simulink library "udp_library"  (Simulink 7.5)
settings: Solver=ode45  StartTime=0.0  StopTime=10.0  RelTol=1e-3
InitFcn:
  | updateAnnotation.m
undefined symbols (not defined in the file): updateAnnotation
settings Model: Creator=paul  LastModifiedBy=paul.liu

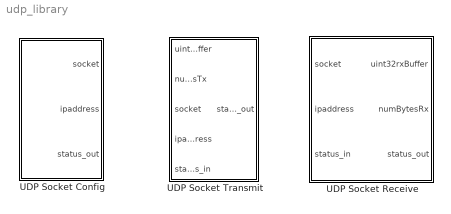
== system udp_library ==
  UDP Socket Config : Subsystem  InitFcn=updateAnnotation();  mask{server_ip='127.0.0.1', server_port=1002, client_ip='127.0.0.1', client_port=1001}
      mask prompts: server_ip "Server IP"; server_port "Server Port"; client_ip "Client IP"; client_port "Client Port"
      settings: AttributesFormatString=Ver 1.0
  UDP Socket Receive : Subsystem  InitFcn=updateAnnotation();
      settings: AttributesFormatString=Ver 1.0
  UDP Socket Transmit : Subsystem  InitFcn=updateAnnotation();
      settings: AttributesFormatString=Ver 1.0

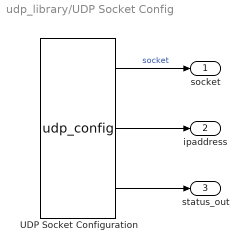
== system udp_library/UDP Socket Config ==
  UDP Socket Configuration : S-Function  FunctionName=udp_config  Parameters=server_ip,server_port,client_ip,client_port  EnableBusSupport=off
  socket : Outport  OutDataType=fixdt(1, 16)  OutScaling=2^0
  ipaddress : Outport  Port=2  OutDataType=fixdt(1, 16)  OutScaling=2^0
  status_out : Outport  Port=3  OutDataType=fixdt(1, 16)  OutScaling=2^0
  wires:
  UDP Socket Configuration/1 -> socket/1  "socket"
  UDP Socket Configuration/2 -> ipaddress/1
  UDP Socket Configuration/3 -> status_out/1

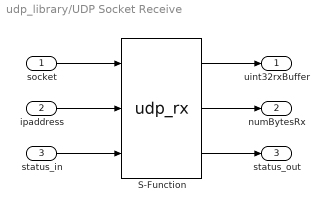
== system udp_library/UDP Socket Receive ==
  socket : Inport  OutDataType=fixdt(1, 16)  OutScaling=2^0
  ipaddress : Inport  Port=2  OutDataType=fixdt(1, 16)  OutScaling=2^0
  status_in : Inport  Port=3  OutDataType=fixdt(1, 16)  OutScaling=2^0
  S-Function : S-Function  FunctionName=udp_rx  EnableBusSupport=off
  uint32rxBuffer : Outport  OutDataType=fixdt(1, 16)  OutScaling=2^0
  numBytesRx : Outport  Port=2  OutDataType=fixdt(1, 16)  OutScaling=2^0
  status_out : Outport  Port=3  OutDataType=fixdt(1, 16)  OutScaling=2^0
  wires:
  S-Function/1 -> uint32rxBuffer/1
  S-Function/2 -> numBytesRx/1
  S-Function/3 -> status_out/1
  socket/1 -> S-Function/1
  ipaddress/1 -> S-Function/2
  status_in/1 -> S-Function/3

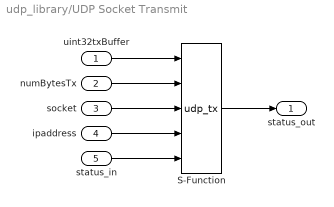
== system udp_library/UDP Socket Transmit ==
  uint32txBuffer : Inport  OutDataType=fixdt(1, 16)  OutScaling=2^0
  numBytesTx : Inport  Port=2  OutDataType=fixdt(1, 16)  OutScaling=2^0
  socket : Inport  Port=3  OutDataType=fixdt(1, 16)  OutScaling=2^0
  ipaddress : Inport  Port=4  OutDataType=fixdt(1, 16)  OutScaling=2^0
  status_in : Inport  Port=5  OutDataType=fixdt(1, 16)  OutScaling=2^0
  S-Function : S-Function  FunctionName=udp_tx  EnableBusSupport=off
  status_out : Outport  OutDataType=fixdt(1, 16)  OutScaling=2^0
  wires:
  status_in/1 -> S-Function/5
  ipaddress/1 -> S-Function/4
  socket/1 -> S-Function/3
  numBytesTx/1 -> S-Function/2
  uint32txBuffer/1 -> S-Function/1
  S-Function/1 -> status_out/1
